simulink model "Intake_Transfer_Function"  (R2022a)
settings: Solver=VariableStepAuto  StartTime=0.0  StopTime=inf  RelTol=1e-3
values from neighbouring files (symbols this model uses):
  ArmatureInductance = 131*10^(-6)    (= 0.000131)    [Intake.m]
  ArmatureResistance = 1.8    [Intake.m]
  DampingConstant = (0.01^2)/1.8    (= 5.55555555556e-05)    [Intake.m]
  kEMF = 0.01    [Intake.m]
  kT = 0.01    [Intake.m]
  LoadAndRotorInertia = LoadInertia+RotorInertia    (= 1.8535689315e-05)    [Intake.m]
settings Model: PacingRate=0.790000  Creator=niksharma  LastModifiedBy=JD Herlehy
settings DebuggingCC: UnconnectedInputMsg=warning  UnconnectedOutputMsg=warning  UnconnectedLineMsg=warning
settings RTWCC: DLArmComputeVersion=19.05

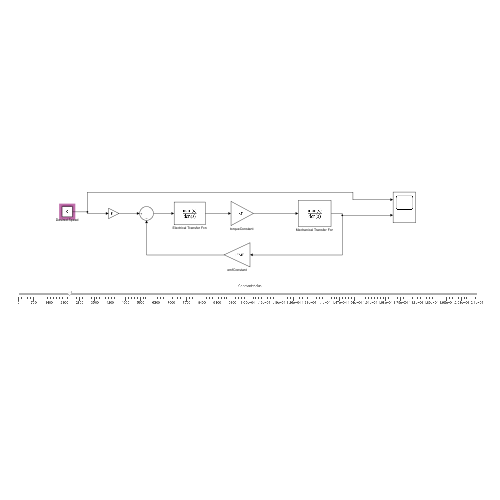
[thumbnail: Simulink's stored preview of the top-level diagram]
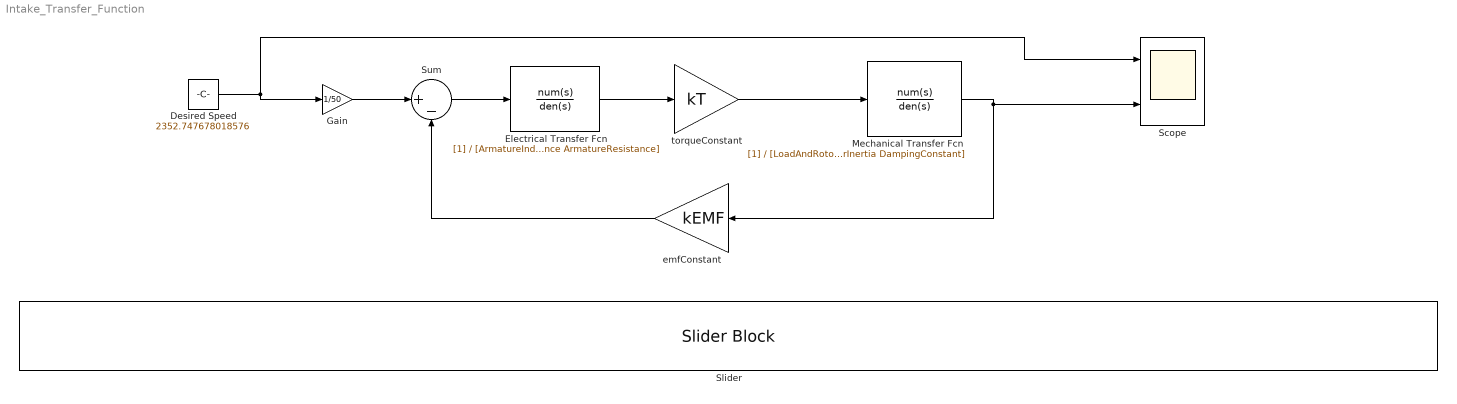
== system Intake_Transfer_Function ==
  Desired Speed : Constant  Value=2352.747678018576
  Electrical Transfer Fcn : TransferFcn  Denominator=[ArmatureInductance ArmatureResistance]
  Gain : Gain  Gain=1/50
  Mechanical Transfer Fcn : TransferFcn  Denominator=[LoadAndRotorInertia DampingConstant]
  Scope : Scope  NumInputPorts=2
  Slider : SliderBlock  ScaleMax=21000
  Sum : Sum  Inputs=|+-
  emfConstant : Gain  Gain=kEMF
  "torqueConstant " : Gain  Gain=kT
  wires:
  Electrical Transfer Fcn/1 -> "torqueConstant "/1
  "torqueConstant "/1 -> Mechanical Transfer Fcn/1
  emfConstant/1 -> Sum/2
  Sum/1 -> Electrical Transfer Fcn/1
  Mechanical Transfer Fcn/1 -> emfConstant/1, Scope/2
  Desired Speed/1 -> Gain/1, Scope/1
  Gain/1 -> Sum/1
